simulink model "HILMODEL_IFBlock_2018"  (R2020b)
settings: Solver=FixedStepAuto  StartTime=0.0  StopTime=30  RelTol=1e-3  EnableMultiTasking=on
libraries: arduinolib x5
settings Model: SILPILModeSetting=veronly  ExtModeTrigDuration=2  Creator=99003188  LastModifiedBy=99003188
settings SolverCC: AutoInsertRateTranBlk=on
settings OptimizationCC: EnhancedBackFolding=on  PassReuseOutputArgsAs=Individual arguments  ZeroExternalMemoryAtStartup=off  ZeroInternalMemoryAtStartup=off  MaxStackSize=64  OptimizeBlockOrder=speed  DifferentSizesBufferReuse=on  OptimizationCustomize=off  EfficientTunableParamExpr=on
settings DebuggingCC: ParameterTunabilityLossMsg=error
settings HardwareCC: ProdBitPerInt=16  ProdBitPerPointer=16  ProdBitPerSizeT=16  ProdBitPerPtrDiffT=16  ProdLargestAtomicFloat=None  ProdWordSize=8  ProdHWDeviceType=Atmel->AVR  UseEmbeddedCoderFeatures=off  UseSimulinkCoderFeatures=off
settings SFSimCC: MATLABDynamicMemAlloc=off
settings RTWCC: Description=Embedded Coder  SystemTargetFile=ert.tlc  HardwareBoard=Arduino Uno  TemplateMakefile=ert_default_tmf  Toolchain=Arduino AVR  BuildConfiguration=Faster Runs
settings CodeAppCC: ForceParamTrailComments=on  IgnoreCustomStorageClasses=off  OperatorAnnotations=on  SimulinkDataObjDesc=on  SFDataObjDesc=on  InsertBlockDesc=on
settings ERTTargetCC: SupportContinuousTime=on  SupportNonInlinedSFcns=on  SupportVariableSizeSignals=on  ExtModeStaticAllocSize=250

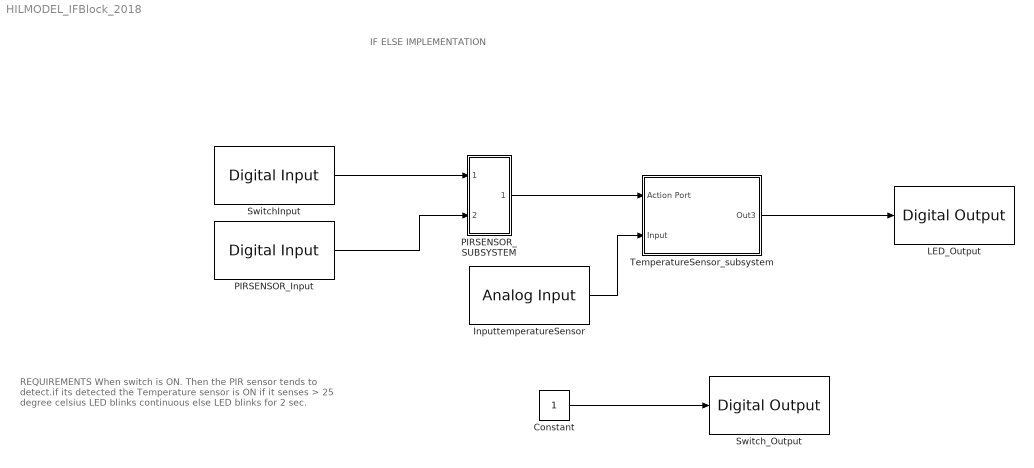
== system HILMODEL_IFBlock_2018 ==
  note: IF ELSE IMPLEMENTATION
  note: REQUIREMENTS
      |
      | When switch is ON. Then the PIR sensor tends to detect.if its detected the Temperature sensor is ON if it senses > 25 degree celsius LED blinks continuous else LED blinks for 2 sec.
  Constant : Constant
  InputtemperatureSensor : arduinolib/Analog Input  pinNumber=4  ReadResultsOnly=off  ConversionTriggerSource=Software  ExternalTriggerType=uint32( 0 )  OutputDataType=uint16  EnableConversionCompleteNotify=off  EnableOuputStatus=off  SampleTime=-1  blockPlatform=arduino
  LED_Output : arduinolib/Digital Output  pinNumber=13  Direction=output  blockPlatform=arduino
  PIRSENSOR_Input : arduinolib/Digital Input  pinNumber=10  mode=Default  Direction=input  SampleTime=0.1  blockPlatform=arduino
  PIRSENSOR_SUBSYSTEM : Subsystem
  SwitchInput : arduinolib/Digital Input  pinNumber=8  mode=Default  Direction=input  SampleTime=0.1  blockPlatform=arduino
  Switch_Output : arduinolib/Digital Output  pinNumber=9  Direction=output  blockPlatform=arduino
  TemperatureSensor_subsystem : Subsystem
  wires:
  Constant/1 -> Switch_Output/1
  SwitchInput/1 -> PIRSENSOR_SUBSYSTEM/1(In1)
  PIRSENSOR_SUBSYSTEM/1(Out2) -> TemperatureSensor_subsystem/1(Action Port)
  TemperatureSensor_subsystem/1(Out3) -> LED_Output/1
  PIRSENSOR_Input/1 -> PIRSENSOR_SUBSYSTEM/2(Input)
  InputtemperatureSensor/1 -> TemperatureSensor_subsystem/2(Input)

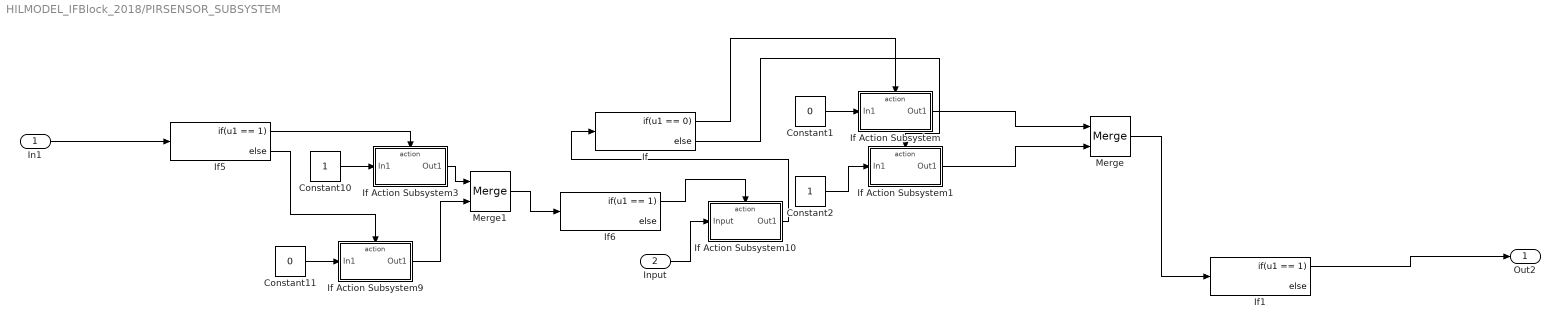
== system HILMODEL_IFBlock_2018/PIRSENSOR_SUBSYSTEM ==
  In1 : Inport
  Input : Inport  Port=2
  Constant1 : Constant  Value=0
  Constant10 : Constant
  Constant11 : Constant  Value=0
  Constant2 : Constant
  If : If  IfExpression=u1 == 0
  If Action Subsystem : Subsystem  TreatAsAtomicUnit=on
  If Action Subsystem1 : Subsystem  TreatAsAtomicUnit=on
  If Action Subsystem10 : Subsystem  TreatAsAtomicUnit=on
  If Action Subsystem3 : Subsystem  TreatAsAtomicUnit=on
  If Action Subsystem9 : Subsystem  TreatAsAtomicUnit=on
  If1 : If  IfExpression=u1 == 1
  If5 : If  IfExpression=u1 == 1
  If6 : If  IfExpression=u1 == 1
  Merge : Merge
  Merge1 : Merge
  Out2 : Outport
  wires:
  Constant1/1 -> If Action Subsystem/1(In1)
  Constant10/1 -> If Action Subsystem3/1(In1)
  If/2 -> If Action Subsystem1/Action
  If Action Subsystem/1(Out1) -> Merge/1
  If/1 -> If Action Subsystem/Action
  Constant11/1 -> If Action Subsystem9/1(In1)
  If5/1 -> If Action Subsystem3/Action
  If Action Subsystem1/1(Out1) -> Merge/2
  If Action Subsystem9/1(Out1) -> Merge1/2
  In1/1 -> If5/1
  If5/2 -> If Action Subsystem9/Action
  Merge1/1 -> If6/1
  Merge/1 -> If1/1
  If6/1 -> If Action Subsystem10/Action
  Constant2/1 -> If Action Subsystem1/1(In1)
  If Action Subsystem3/1(Out1) -> Merge1/1
  If Action Subsystem10/1(Out1) -> If/1
  If1/1 -> Out2/1
  Input/1 -> If Action Subsystem10/1(Input)

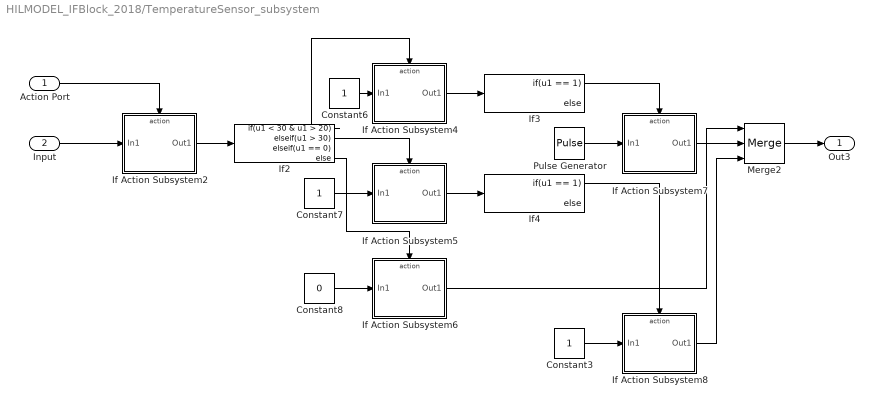
== system HILMODEL_IFBlock_2018/TemperatureSensor_subsystem ==
  Action Port : Inport
  Input : Inport  Port=2
  Constant3 : Constant
  Constant6 : Constant
  Constant7 : Constant
  Constant8 : Constant  Value=0
  If Action Subsystem2 : Subsystem  TreatAsAtomicUnit=on
  If Action Subsystem4 : Subsystem  TreatAsAtomicUnit=on
  If Action Subsystem5 : Subsystem  TreatAsAtomicUnit=on
  If Action Subsystem6 : Subsystem  TreatAsAtomicUnit=on
  If Action Subsystem7 : Subsystem  TreatAsAtomicUnit=on
  If Action Subsystem8 : Subsystem  TreatAsAtomicUnit=on
  If2 : If  IfExpression=u1 < 30 & u1 > 20  ElseIfExpressions=u1 > 30,u1 == 0
  If3 : If  IfExpression=u1 == 1
  If4 : If  IfExpression=u1 == 1
  Merge2 : Merge  Inputs=3
  Pulse Generator : DiscretePulseGenerator  PulseType=Time based  PulseWidth=50
  Out3 : Outport
  wires:
  Merge2/1 -> Out3/1
  If2/1 -> If Action Subsystem4/Action
  Action Port/1 -> If Action Subsystem2/Action
  If2/4 -> If Action Subsystem6/Action
  If Action Subsystem6/1(Out1) -> Merge2/1
  Input/1 -> If Action Subsystem2/1(In1)
  If Action Subsystem2/1(Out1) -> If2/1
  Pulse Generator/1 -> If Action Subsystem7/1(In1)
  Constant7/1 -> If Action Subsystem5/1(In1)
  Constant3/1 -> If Action Subsystem8/1(In1)
  If Action Subsystem4/1(Out1) -> If3/1
  If Action Subsystem8/1(Out1) -> Merge2/3
  Constant8/1 -> If Action Subsystem6/1(In1)
  If Action Subsystem7/1(Out1) -> Merge2/2
  If4/1 -> If Action Subsystem8/Action
  If Action Subsystem5/1(Out1) -> If4/1
  Constant6/1 -> If Action Subsystem4/1(In1)
  If3/1 -> If Action Subsystem7/Action
  If2/2 -> If Action Subsystem5/Action

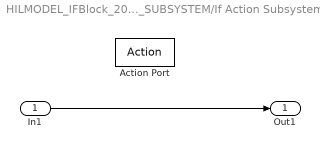
== system HILMODEL_IFBlock_2018/PIRSENSOR_SUBSYSTEM/If Action Subsystem ==
  In1 : Inport
  Action Port : ActionPort  ActionPortLabel=if(u1 == 0)
  Out1 : Outport
  wires:
  In1/1 -> Out1/1

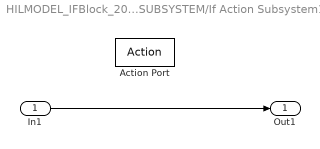
== system HILMODEL_IFBlock_2018/PIRSENSOR_SUBSYSTEM/If Action Subsystem1 ==
  In1 : Inport
  Action Port : ActionPort  ActionPortLabel=else
  Out1 : Outport
  wires:
  In1/1 -> Out1/1

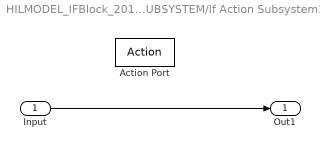
== system HILMODEL_IFBlock_2018/PIRSENSOR_SUBSYSTEM/If Action Subsystem10 ==
  Input : Inport
  Action Port : ActionPort  ActionPortLabel=if(u1 == 1)
  Out1 : Outport
  wires:
  Input/1 -> Out1/1

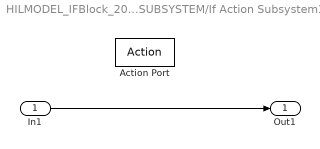
== system HILMODEL_IFBlock_2018/PIRSENSOR_SUBSYSTEM/If Action Subsystem3 ==
  In1 : Inport
  Action Port : ActionPort  ActionPortLabel=if(u1 == 1)
  Out1 : Outport
  wires:
  In1/1 -> Out1/1

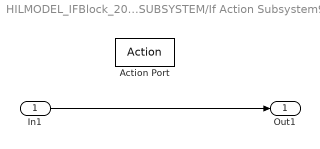
== system HILMODEL_IFBlock_2018/PIRSENSOR_SUBSYSTEM/If Action Subsystem9 ==
  In1 : Inport
  Action Port : ActionPort  ActionPortLabel=else
  Out1 : Outport
  wires:
  In1/1 -> Out1/1

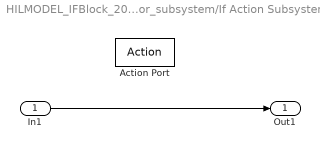
== system HILMODEL_IFBlock_2018/TemperatureSensor_subsystem/If Action Subsystem2 ==
  In1 : Inport
  Action Port : ActionPort  ActionPortLabel=if(u1 == 1)
  Out1 : Outport
  wires:
  In1/1 -> Out1/1

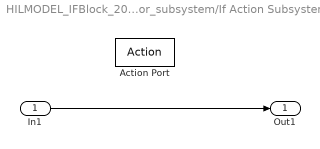
== system HILMODEL_IFBlock_2018/TemperatureSensor_subsystem/If Action Subsystem4 ==
  In1 : Inport
  Action Port : ActionPort  ActionPortLabel=if(u1 < 30 & u1 > 20)
  Out1 : Outport
  wires:
  In1/1 -> Out1/1

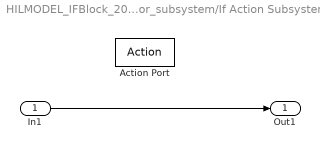
== system HILMODEL_IFBlock_2018/TemperatureSensor_subsystem/If Action Subsystem5 ==
  In1 : Inport
  Action Port : ActionPort  ActionPortLabel=elseif(u1 > 30)
  Out1 : Outport
  wires:
  In1/1 -> Out1/1

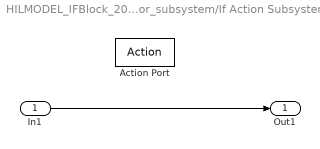
== system HILMODEL_IFBlock_2018/TemperatureSensor_subsystem/If Action Subsystem6 ==
  In1 : Inport
  Action Port : ActionPort  ActionPortLabel=else
  Out1 : Outport
  wires:
  In1/1 -> Out1/1

== system HILMODEL_IFBlock_2018/TemperatureSensor_subsystem/If Action Subsystem7 ==
  In1 : Inport
  Action Port : ActionPort  ActionPortLabel=if(u1 == 1)
  Out1 : Outport
  wires:
  In1/1 -> Out1/1

== system HILMODEL_IFBlock_2018/TemperatureSensor_subsystem/If Action Subsystem8 ==
  In1 : Inport
  Action Port : ActionPort  ActionPortLabel=if(u1 == 1)
  Out1 : Outport
  wires:
  In1/1 -> Out1/1
